simulink model "PID_Controller"  (R2020b)
settings: Solver=VariableStepAuto  StartTime=0.0  StopTime=0.2  RelTol=1e-3
undefined symbols (not defined in the file or in its folder): Kd, Ki, Kp
settings Model: DataDictionary=Problem4.sldd  Creator=Shirish  LastModifiedBy=Shirish
settings DataIOCC: SaveOutput=off  SaveTime=off

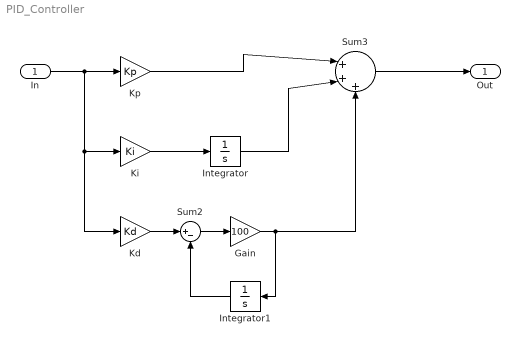
== system PID_Controller ==
  In : Inport  OutDataTypeStr=double  PortDimensions=1  SampleTime=0
  Gain : Gain  Gain=100
  Integrator : Integrator
  Integrator1 : Integrator
  Kd : Gain  Gain=Kd
  Ki : Gain  Gain=Ki
  Kp : Gain  Gain=Kp
  Sum2 : Sum  Inputs=|+-
  Sum3 : Sum  Inputs=|+++
  Out : Outport  OutDataTypeStr=double  PortDimensions=1  SampleTime=0
  wires:
  Gain/1 -> Integrator1/1, Sum3/3
  Sum2/1 -> Gain/1
  In/1 -> Kp/1, Kd/1, Ki/1
  Kp/1 -> Sum3/1
  Integrator/1 -> Sum3/2
  Sum3/1 -> Out/1
  Kd/1 -> Sum2/1
  Integrator1/1 -> Sum2/2
  Ki/1 -> Integrator/1
